simulink model "SPMSM_simul"  (R2021a)
settings: Solver=VariableStepAuto  StartTime=0.0  StopTime=0.5  RelTol=1e-3
values from neighbouring files (symbols this model uses):
  F = [-Rs/Lq -(Pol*Lamb)/(2*Lq) 0; (3*Pol*Lamb)/(2*2*Jm) -Bm/Jm 0; 0 1 0]    [SPMSM.m]
  G = [1/Lq ;0 ;0]    [SPMSM.m]
  H = [0 0 1]    [SPMSM.m]
  K = acker(F,G,p)    [SPMSM.m]
  K1_integ = K_temp_integ(1)    [SPMSM.m]
  K1_integ_NSRL = K_temp_integ_NSRL(1)    [SPMSM.m]
  K_integ = [K_temp_integ(2) K_temp_integ(3) K_temp_integ(4)]    [SPMSM.m]
  K_integ_NSRL = [K_temp_integ_NSRL(2) K_temp_integ_NSRL(3) K_temp_integ_NSRL(4)]    [SPMSM.m]
  K_lqr = acker(F,G,lqr_pole)    [SPMSM.m]
  L = L'    [SPMSM.m]
  L_lqr = L_lqr'    [SPMSM.m]
  N_bar = Nu + K*Nx    [SPMSM.m]
  N_lqr_bar = Nu + K_lqr*Nx    [SPMSM.m]
  r = 1    [SPMSM.m]
libraries: simulink x5
settings Model: Creator=syl12  LastModifiedBy=syl12

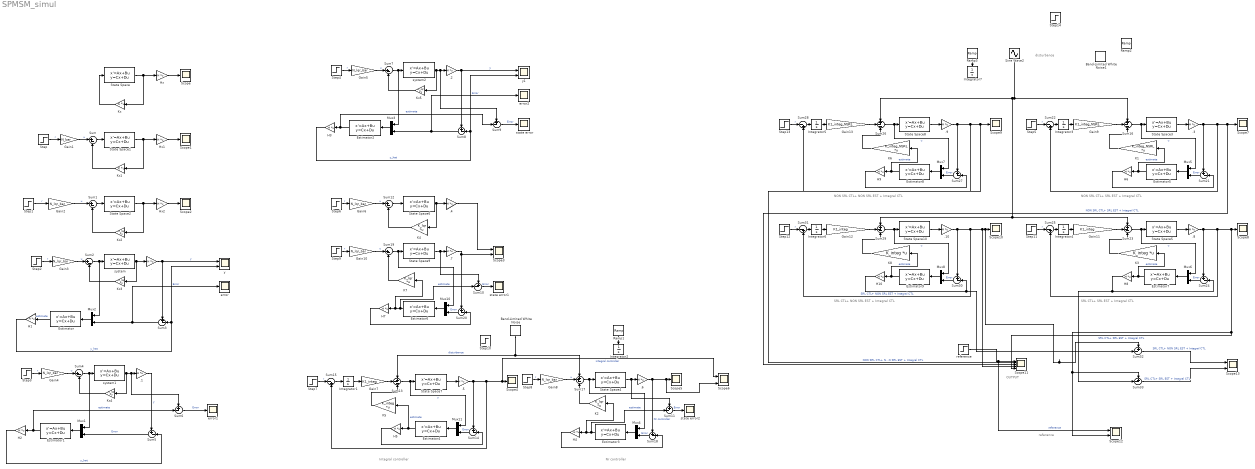
== system SPMSM_simul ==
  note: reference
  note: disturbance
  note: Integral controller
  note: Nr controller
  note: NON SRL CTL+ SRL EST + Integral CTL
  note: SRL CTL+ SRL EST + Integral CTL
  note: NON SRL CTL+ NON SRL EST + Integral CTL
  note: SRL CTL+ NON SRL EST + Integral CTL
  note: OUTPUT
  .{,1..10} (11 alike) : Gain  Gain=H  Multiplication=Matrix(K*u)
  Band-Limited White Noise : simulink/Sources/Band-Limited White Noise  Cov=[0.100]  Ts=0.0001  seed=[23341]
  Band-Limited White Noise1 : simulink/Sources/Band-Limited White Noise  Cov=[0.100]  Ts=0.0001  seed=[23341]
  Estimator{,1,7..8} (4 alike) : StateSpace  A=F  B=[G L]  C=eye(3)  D=zeros(3,2)  InitialCondition=[1 0 0]
  Estimator{2..3,5..6,9} (5 alike) : StateSpace  A=F  B=[G L_lqr]  C=eye(3)  D=zeros(3,2)  InitialCondition=[1 0 0]
  Estimator4 : StateSpace  A=F  B=[G L_lqr]  C=eye(3)  D=zeros(3,2)  InitialCondition=[0 0 0]
  Gain1 : Gain  Gain=N_bar
  Gain{2..6,8,10} (7 alike) : Gain  Gain=N_lqr_bar
  Gain11 : Gain  Gain=K1_integ
  Gain12 : Gain  Gain=K1_integ
  Gain13 : Gain  Gain=K1_integ_NSRL
  Gain7 : Gain  Gain=K1_integ
  Gain9 : Gain  Gain=K1_integ_NSRL
  H{1..10} (10 alike) : Gain  Gain=H  Multiplication=Matrix(K*u)
  Hx : Gain  Gain=H  Multiplication=Matrix(K*u)
  Hx1 : Gain  Gain=H  Multiplication=Matrix(K*u)
  Hx2 : Gain  Gain=H  Multiplication=Matrix(K*u)
  Integrator{1..7} (7 alike) : Integrator
  K1 : Gain  Gain=K_integ_NSRL  Multiplication=Matrix(K*u)
  K2 : Gain  Gain=K_lqr  Multiplication=Matrix(K*u)
  K3 : Gain  Gain=K_integ  Multiplication=Matrix(K*u)
  K4 : Gain  Gain=K_lqr  Multiplication=Matrix(K*u)
  K5 : Gain  Gain=K_integ  Multiplication=Matrix(K*u)
  K6 : Gain  Gain=K_integ_NSRL  Multiplication=Matrix(K*u)
  K7 : Gain  Gain=K_lqr  Multiplication=Matrix(K*u)
  K8 : Gain  Gain=K_integ  Multiplication=Matrix(K*u)
  Kx : Gain  Gain=K  Multiplication=Matrix(K*u)
  Kx1 : Gain  Gain=K  Multiplication=Matrix(K*u)
  Kx{2..5} (4 alike) : Gain  Gain=K_lqr  Multiplication=Matrix(K*u)
  Mux{1..8,10..11} (10 alike) : Mux  Inputs=2
  Ramp1 : simulink/Sources/Ramp  slope=10000  start=0.15  InitialOutput=0
  Ramp2 : simulink/Sources/Ramp  slope=1000  start=0.15  InitialOutput=0
  Ramp3 : simulink/Sources/Ramp  slope=1000  start=0.15  InitialOutput=0
  Scope{,1..2,4..5,7..10} (9 alike) : Scope
  Scope11 : Scope  NumInputPorts=5
  Scope{3,6,12..13} (4 alike) : Scope  NumInputPorts=2
  Sine Wave2 : Sin  Amplitude=100  Frequency=1000  SampleTime=0
  State Space : StateSpace  A=F  B=G  C=eye(3)  D=zeros(3,1)  InitialCondition=-1
  State Space1 : StateSpace  A=F  B=G  C=eye(3)  D=zeros(3,1)  InitialCondition=0
  State Space{3..5,8..10} (6 alike) : StateSpace  A=F  B=G  C=eye(3)  D=zeros(3,1)  InitialCondition=[0 0 0]
  State Space2 : StateSpace  A=F  B=G  C=eye(3)  D=zeros(3,1)  InitialCondition=0
  State Space6 : StateSpace  A=F  B=G  C=eye(3)  D=zeros(3,1)  InitialCondition=[0.3 0 0]
  State Space7 : StateSpace  A=F  B=G  C=eye(3)  D=zeros(3,1)  InitialCondition=[0.3 0 0]
  Step{,1..4,6,8..9} (8 alike) : Step  Time=0  After=r  SampleTime=0
  Step10 : Step  Time=0.15  After=10  SampleTime=0
  Step{5,7,11..13} (5 alike) : Step  Time=0  Before=1  SampleTime=0
  Step14 : Step  Time=0.15  After=10  SampleTime=0
  Sum{,1..2,4,7,12,19} (7 alike) : Sum  Inputs=|+-
  Sum{3,5..6,8..11,14,18,20..21,24,27,30,32..33} (16 alike) : Sum  Inputs=+-|
  Sum{13,16,23,26,29} (5 alike) : Sum  Inputs=+--
  Sum{15,22,25,28,31} (5 alike) : Sum  Inputs=|-+
  Sum17 : Sum  Inputs=++-
  error : Scope
  error1 : Scope
  error2 : Scope
  reference : Step  Time=0  Before=1  SampleTime=0
  state error : Scope
  state error1 : Scope
  state error2 : Scope
  system : StateSpace  A=F  B=G  C=eye(3)  D=zeros(3,1)  InitialCondition=[0 0 0]
  system1 : StateSpace  A=F  B=G  C=eye(3)  D=zeros(3,1)  InitialCondition=[0 0 0]
  system2 : StateSpace  A=F  B=G  C=eye(3)  D=zeros(3,1)  InitialCondition=[0 0 0]
  y : Scope  NumInputPorts=2
  y1 : Scope  NumInputPorts=2
  wires:
  State Space/1 -> Kx/1, Hx/1
  Kx/1 -> State Space/1
  Hx/1 -> Scope/1
  Step/1 -> Gain1/1  "r"
  Hx1/1 -> Scope1/1
  Kx1/1 -> Sum/2
  State Space1/1 -> Kx1/1, Hx1/1
  Sum/1 -> State Space1/1
  Gain1/1 -> Sum/1  "u"
  State Space2/1 -> Kx2/1, Hx2/1
  Sum1/1 -> State Space2/1
  Step1/1 -> Gain2/1  "r"
  Hx2/1 -> Scope2/1
  Gain2/1 -> Sum1/1  "u"
  Kx2/1 -> Sum1/2
  ./1 -> y/1, Sum3/1  "y"
  Kx3/1 -> Sum2/2
  Mux2/1 -> Estimator/1
  Sum3/1 -> error/1, Mux2/2  "Error"
  Step2/1 -> Gain3/1  "r"
  Sum2/1 -> Mux2/1, system/1
  system/1 -> Kx3/1, ./1
  Gain3/1 -> Sum2/1  "u"
  H1/1 -> y/2, Sum3/2  "y_hat"
  Estimator/1 -> H1/1  "estimate"
  Sum4/1 -> Mux1/1, system1/1
  Sum5/1 -> Mux1/2  "Error"
  .1/1 -> Sum5/1  "y"
  H2/1 -> Sum5/2  "y_hat"
  system1/1 -> Kx4/1, Sum6/1, .1/1
  Kx4/1 -> Sum4/2
  Step3/1 -> Gain4/1  "r"
  Gain4/1 -> Sum4/1  "u"
  Mux1/1 -> Estimator1/1
  Estimator1/1 -> Sum6/2, H2/1  "estimate"
  Sum6/1 -> error1/1  "Error"
  H3/1 -> y1/2, Sum8/2  "y_hat"
  Estimator2/1 -> Sum9/2, H3/1  "estimate"
  Sum8/1 -> error2/1, Mux3/2  "Error"
  Step4/1 -> Gain5/1  "r"
  Mux3/1 -> Estimator2/1
  Gain5/1 -> Sum7/1  "u"
  .2/1 -> y1/1, Sum8/1  "y"
  Sum7/1 -> Mux3/1, system2/1
  Kx5/1 -> Sum7/2
  system2/1 -> Kx5/1, Sum9/1, .2/1
  Sum9/1 -> state error/1  "Error"
  State Space9/1 -> Sum10/1, .7/1
  Sum20/1 -> Mux10/2  "Error"
  Sum19/1 -> Mux10/1, State Space9/1
  Step6/1 -> Gain6/1  "r"
  Sum12/1 -> State Space6/1
  K4/1 -> Sum12/2
  Gain6/1 -> Sum12/1  "u"
  State Space6/1 -> .4/1, K4/1
  H7/1 -> Sum20/2
  Gain10/1 -> Sum19/1  "u"
  Step9/1 -> Gain10/1  "r"
  K7/1 -> Sum19/2
  Estimator6/1 -> Sum10/2, K7/1, H7/1  "estimate"
  Mux10/1 -> Estimator6/1
  .7/1 -> Scope3/2, Sum20/1
  Sum10/1 -> state error1/1  "Error"
  .4/1 -> Scope3/1
  State Space7/1 -> .5/1
  Sum13/1 -> Mux11/1, State Space7/1  "u"
  Sum14/1 -> Mux11/2  "Error"
  H5/1 -> Sum14/2
  Sum15/1 -> Integrator1/1
  Mux11/1 -> Estimator4/1
  Step7/1 -> Sum15/1  "r"
  Estimator4/1 -> H5/1, K5/1  "estimate"
  .5/1 -> Scope6/1, Scope4/1, Sum15/2, Sum14/1  "integral controller"
  Integrator1/1 -> Gain7/1
  Gain7/1 -> Sum13/2
  K5/1 -> Sum13/3
  Band-Limited White Noise/1 -> Sum13/1, Sum17/1  "disturbance"
  H4/1 -> Sum18/2
  Mux4/1 -> Estimator3/1
  Sum11/1 -> state error2/1  "Error"
  .6/1 -> Sum18/1, Scope6/2, Scope5/1  "Nr controller"
  Sum17/1 -> Mux4/1, State Space4/1
  Estimator3/1 -> Sum11/2, K2/1, H4/1  "estimate"
  Step8/1 -> Gain8/1  "r"
  Sum18/1 -> Mux4/2  "Error"
  State Space4/1 -> Sum11/1, .6/1
  Gain8/1 -> Sum17/2  "u"
  K2/1 -> Sum17/3
  Ramp1/1 -> Integrator2/1
  Mux5/1 -> Estimator5/1
  Integrator3/1 -> Gain9/1
  .3/1 -> Scope11/3, Scope7/1, Sum22/2, Sum21/1  "NON SRL CTL+ SRL EST + Integral CTL"
  Step5/1 -> Sum22/1  "r"
  Sum21/1 -> Mux5/2  "Error"
  Estimator5/1 -> K1/1, H6/1  "estimate"
  State Space3/1 -> .3/1
  H6/1 -> Sum21/2
  Sum22/1 -> Integrator3/1
  Sum16/1 -> Mux5/1, State Space3/1  "u"
  Step11/1 -> Sum25/1  "r"
  .8/1 -> Sum33/1, Scope12/2, Scope11/5, Scope8/1, Sum25/2, Sum24/1  "SRL CTL+ SRL EST + Integral CTL"
  Integrator4/1 -> Gain11/1
  Mux6/1 -> Estimator7/1
  Sum25/1 -> Integrator4/1
  Sum23/1 -> Mux6/1, State Space5/1  "u"
  H8/1 -> Sum24/2, Sum33/2
  Estimator7/1 -> K3/1, H8/1  "estimate"
  State Space5/1 -> .8/1
  Sum24/1 -> Mux6/2  "Error"
  Step13/1 -> Sum28/1  "r"
  .9/1 -> Scope11/2, Scope9/1, Sum28/2, Sum27/1  "NON SRL CTL+ NON SRL EST + Integral CTL"
  Mux7/1 -> Estimator8/1
  Sum28/1 -> Integrator5/1
  Sum26/1 -> Mux7/1, State Space8/1  "u"
  State Space8/1 -> .9/1
  Sum27/1 -> Mux7/2  "Error"
  Step12/1 -> Sum31/1  "r"
  Integrator5/1 -> Gain13/1
  Sum30/1 -> Mux8/2  "Error"
  State Space10/1 -> .10/1
  Estimator9/1 -> K8/1, H10/1  "estimate"
  H10/1 -> Sum32/2, Sum30/2
  Integrator6/1 -> Gain12/1
  Mux8/1 -> Estimator9/1
  .10/1 -> Scope11/4, Sum32/1, Scope10/1, Sum31/2, Sum30/1  "SRL CTL+ NON SRL EST + Integral CTL"
  Estimator8/1 -> K6/1, H9/1  "estimate"
  Sum31/1 -> Integrator6/1
  Sum29/1 -> Mux8/1, State Space10/1  "u"
  H9/1 -> Sum27/2
  K8/1 -> Sum29/3
  Gain12/1 -> Sum29/2
  Gain13/1 -> Sum26/2
  K6/1 -> Sum26/3
  Gain9/1 -> Sum16/2
  K1/1 -> Sum16/3
  K3/1 -> Sum23/3
  Gain11/1 -> Sum23/2
  reference/1 -> Scope11/1, Scope12/1  "reference"
  Sine Wave2/1 -> Sum23/1, Sum29/1, Sum26/1, Sum16/1
  Sum32/1 -> Scope13/1  "SRL CTL+ NON SRL EST + Integral CTL"
  Sum33/1 -> Scope13/2  "SRL CTL+ SRL EST + Integral CTL"
  Ramp3/1 -> Integrator7/1
